simulink model "simulinkTarea1_C20259"  (R2023b)
settings: Solver=ode4  StartTime=0.0  StopTime=31  FixedStep=1e-4  RelTol=1e-3
settings Model: Creator=daas0  LastModifiedBy=daas0

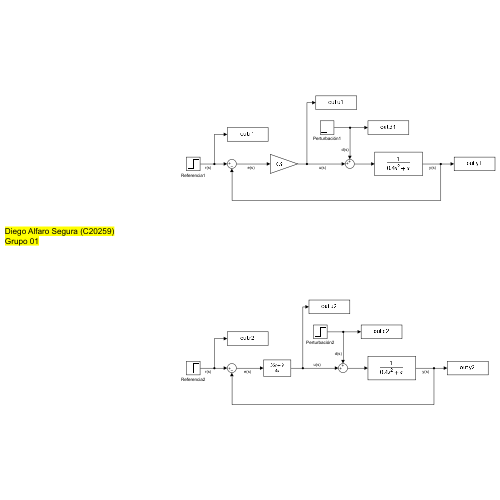
[thumbnail: Simulink's stored preview of the top-level diagram]
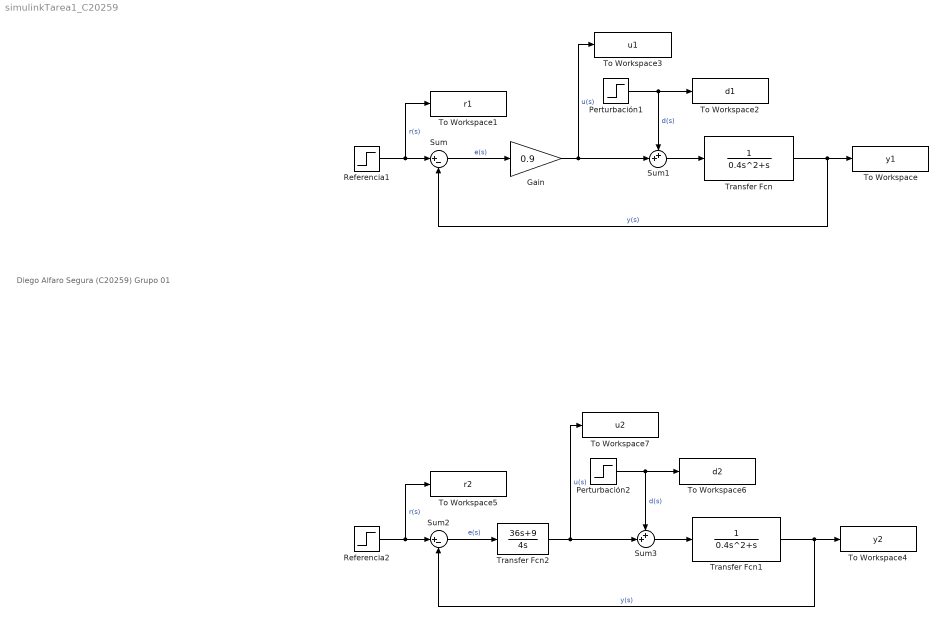
== system simulinkTarea1_C20259 ==
  note: Diego Alfaro Segura (C20259)
      | Grupo 01
  Gain : Gain  Gain=0.9
  Perturbación1 : Step  Time=16  SampleTime=0
  Perturbación2 : Step  Time=16  SampleTime=0
  Referencia1 : Step  SampleTime=0
  Referencia2 : Step  SampleTime=0
  Sum : Sum  Inputs=|+-
  Sum1 : Sum  Inputs=++|
  Sum2 : Sum  Inputs=|+-
  Sum3 : Sum  Inputs=++|
  To Workspace : ToWorkspace  VariableName=y1  SaveFormat=Timeseries  SampleTime=-1
  To Workspace1 : ToWorkspace  VariableName=r1  SaveFormat=Timeseries  SampleTime=-1
  To Workspace2 : ToWorkspace  VariableName=d1  SaveFormat=Timeseries  SampleTime=-1
  To Workspace3 : ToWorkspace  VariableName=u1  SaveFormat=Timeseries  SampleTime=-1
  To Workspace4 : ToWorkspace  VariableName=y2  SaveFormat=Timeseries  SampleTime=-1
  To Workspace5 : ToWorkspace  VariableName=r2  SaveFormat=Timeseries  SampleTime=-1
  To Workspace6 : ToWorkspace  VariableName=d2  SaveFormat=Timeseries  SampleTime=-1
  To Workspace7 : ToWorkspace  VariableName=u2  SaveFormat=Timeseries  SampleTime=-1
  Transfer Fcn : TransferFcn  Denominator=[0.4 1 0]
  Transfer Fcn1 : TransferFcn  Denominator=[0.4 1 0]
  Transfer Fcn2 : TransferFcn  Numerator=[36 9]  Denominator=[4 0]
  wires:
  Referencia1/1 -> To Workspace1/1, Sum/1  "r(s)"
  Sum/1 -> Gain/1  "e(s)"
  Gain/1 -> Sum1/2, To Workspace3/1  "u(s)"
  Sum1/1 -> Transfer Fcn/1
  Transfer Fcn/1 -> Sum/2, To Workspace/1  "y(s)"
  Perturbación1/1 -> To Workspace2/1, Sum1/1  "d(s)"
  Transfer Fcn1/1 -> Sum2/2, To Workspace4/1  "y(s)"
  Sum3/1 -> Transfer Fcn1/1
  Sum2/1 -> Transfer Fcn2/1  "e(s)"
  Transfer Fcn2/1 -> To Workspace7/1, Sum3/2  "u(s)"
  Perturbación2/1 -> To Workspace6/1, Sum3/1  "d(s)"
  Referencia2/1 -> To Workspace5/1, Sum2/1  "r(s)"
